simulink model "predictionModuleTest"  (R2026a)
settings: Solver=VariableStepAuto  StopTime=247  FixedStep=1
settings Model: Creator=hp  LastModifiedBy=hp

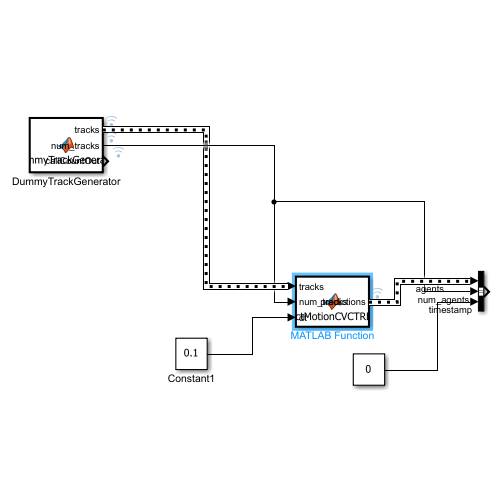
[thumbnail: Simulink's stored preview of the top-level diagram]
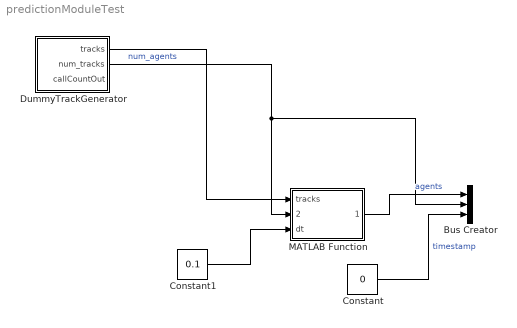
== system predictionModuleTest ==
  Bus Creator : BusCreator  Inputs=3  OutDataTypeStr=Bus: SihPredictionBus
  Constant : Constant  Value=0
  Constant1 : Constant  Value=0.1
  DummyTrackGenerator : MATLAB Function  TreatAsAtomicUnit=on  SystemSampleTime=1
  MATLAB Function : MATLAB Function  TreatAsAtomicUnit=on
  wires:
  DummyTrackGenerator/2(num_tracks) -> Bus Creator/2, MATLAB Function/2(num_tracks)  "num_agents"
  Constant1/1 -> MATLAB Function/3(dt)
  DummyTrackGenerator/1(tracks) -> MATLAB Function/1(tracks)
  MATLAB Function/1(predictions) -> Bus Creator/1  "agents"
  Constant/1 -> Bus Creator/3  "timestamp"

== matlab function predictionModuleTest/DummyTrackGenerator ==
  data: tracks output Bus: SihTrackBus size=40; num_tracks output uint32; callCountOut output
function [tracks, num_tracks, callCountOut] = DummyTrackGenerator() %#codegen
%DUMMYTRACKGENERATOR Loads one real frame from M1's exported data,
% padded to MAX_TRACKS since M1's export is variable-length per frame.

MAX_TRACKS = 40;

persistent perceptionData callCount
if isempty(perceptionData)
    S = coder.load('m1_perception_day4.mat', 'perceptionData');
    perceptionData = S.perceptionData;
    callCount = 0;
end
callCount = callCount + 1;
frameIdx = min(callCount, numel(perceptionData.signals.values));

rawTracks = perceptionData.signals.values(frameIdx).tracks;
n = numel(rawTracks);

invalidTrack = struct( ...
    'id', uint32(0), ...
    'class', AgentClass.Unknown, ...
    'x', 0, ...
    'y', 0, ...
    'heading', 0, ...
    'velocity', 0, ...
    'covariance', zeros(4,4), ...
    'valid', false);

tracks = repmat(invalidTrack, MAX_TRACKS, 1);
for k = 1:min(n, MAX_TRACKS)
    tracks(k) = rawTracks(k);
end

num_tracks = uint32(min(n, MAX_TRACKS));
callCountOut = callCount;
end

== matlab function predictionModuleTest/MATLAB Function ==
  data: tracks input Bus: SihTrackBus size=40; predictions output Bus: SihPredictedAgentBus size=40; num_tracks input uint32; dt input double size=1
function predictions = predictMotionCVCTRBlock(tracks, num_tracks, dt) %#codegen
MAX_TRACKS = 40;
N = 20;
uncertaintyParams = classUncertaintyParams();

persistent prevHeading prevId hasHistory
if isempty(prevHeading)
    prevHeading = zeros(1, MAX_TRACKS);
    prevId = zeros(1, MAX_TRACKS, 'uint32');
    hasHistory = false(1, MAX_TRACKS);
end

predictions = repmat(struct( ...
    'id', uint32(0), ...
    'predicted_positions', zeros(N, 2), ...
    'uncertainty_radius', zeros(N, 1), ...
    'valid', false), MAX_TRACKS, 1);

for i = 1:MAX_TRACKS
    if i > num_tracks || ~tracks(i).valid
        continue
    end
    trk = tracks(i);
    yawRate = 0;
    if hasHistory(i) && prevId(i) == trk.id
        headingDiff = mod(double(trk.heading) - prevHeading(i) + pi, 2*pi) - pi;
        if abs(headingDiff) > 1e-3
            yawRate = headingDiff / dt;
        end
    end
    prevHeading(i) = double(trk.heading);
    prevId(i) = trk.id;
    hasHistory(i) = true;
    [alpha, growthExponent, r0fallback] = lookupClassParams(uncertaintyParams, trk.class);
    pos = zeros(N, 2);
    rad = zeros(N, 1);
    x0 = double(trk.x); y0 = double(trk.y); h0 = double(trk.heading); v = double(trk.velocity);
    r0 = baseUncertaintyRadius(trk.covariance, r0fallback);
    if abs(h0) < 1e-9 && abs(v) < 1e-9
        r0 = r0 * 2;
    end
    for k = 1:N
        t = k * dt;
        if abs(yawRate) > 1e-6
            theta_k = h0 + yawRate * t;
            x_k = x0 + (v / yawRate) * (sin(theta_k) - sin(h0));
            y_k = y0 - (v / yawRate) * (cos(theta_k) - cos(h0));
        else
            x_k = x0 + v * cos(h0) * t;
            y_k = y0 + v * sin(h0) * t;
        end
        pos(k, :) = [x_k, y_k];
        if growthExponent == 1
            rad(k) = r0 + alpha * t;
        else
            rad(k) = r0 + alpha * (t ^ growthExponent);
        end
    end
    predictions(i).id = trk.id;
    predictions(i).predicted_positions = pos;
    predictions(i).uncertainty_radius = rad;
    predictions(i).valid = true;
end
end

function [alpha, growthExponent, r0] = lookupClassParams(uncertaintyParams, agentClass)
alpha = 0; growthExponent = 1; r0 = 0;
found = false;
for k = 1:numel(uncertaintyParams)
    if uncertaintyParams(k).agentClass == agentClass
        alpha = uncertaintyParams(k).alpha;
        growthExponent = uncertaintyParams(k).growthExponent;
        r0 = uncertaintyParams(k).r0;
        found = true;
        break
    end
end
if ~found
    for k = 1:numel(uncertaintyParams)
        if uncertaintyParams(k).agentClass == AgentClass.Pedestrian
            alpha = uncertaintyParams(k).alpha;
            growthExponent = uncertaintyParams(k).growthExponent;
            r0 = uncertaintyParams(k).r0;
            break
        end
    end
end
end

function r0 = baseUncertaintyRadius(covariance, fallback)
P = double(covariance(1:2, 1:2));
if any(isnan(P(:))) || any(isinf(P(:)))
    r0 = fallback;
    return
end
eigVals = real(eig((P + P.') / 2));
maxEig = max(eigVals);
if maxEig <= 0
    r0 = fallback;
else
    r0 = sqrt(maxEig);
end
r0 = real(r0);
end
